simulink model "ExampleMotive"  (Simulink 8.5)
settings: Solver=ode1  StartTime=0.0  StopTime=inf  FixedStep=0.002  RelTol=1e-3
InitFcn:
  | fig_h = figure;
  | ax_h = axes;
  | set(ax_h,'Xlim',[-100 100],'YLim',[-100 100])
settings Model: Creator=adm-drone  LastModifiedBy=jitesh_esb201  ExtModeTrigDuration=5000
settings SolverCC: PositivePriorityOrder=on
settings DataIOCC: SignalLoggingSaveFormat=Dataset
settings OptimizationCC: ExpressionDepthLimit=128
settings DebuggingCC: SolverPrmCheckMsg=warning  FcnCallInpInsideContextMsg=EnableAllAsError
settings RTWCC: SystemTargetFile=quarc_win64.tlc  TemplateMakefile=quarc_default_tmf  Description=QUARC Win64 Target
settings STFCustomTargetCC: TargetPreCompLibLocation=C:\PROGRA~3\QUARC\lib\2013a\win64\release  GeneratePreprocessorConditionals=Disable all  CombineOutputUpdateFcns=on  CPPClassGenCompliant=on  GRTInterface=off  SystemTargetFile=quarc_win64.tlc
settings GRTTargetCC: TargetPreCompLibLocation=C:\PROGRA~3\QUARC\lib\2013a\win64\release  ParMdlRefBuildCompliant=off  CompOptLevelCompliant=off  ConcurrentExecutionCompliant=off  CombineOutputUpdateFcns=on  MatFileLogging=off  GRTInterface=off  ExtMode=on  ExtModeMexFile=quarc_comm

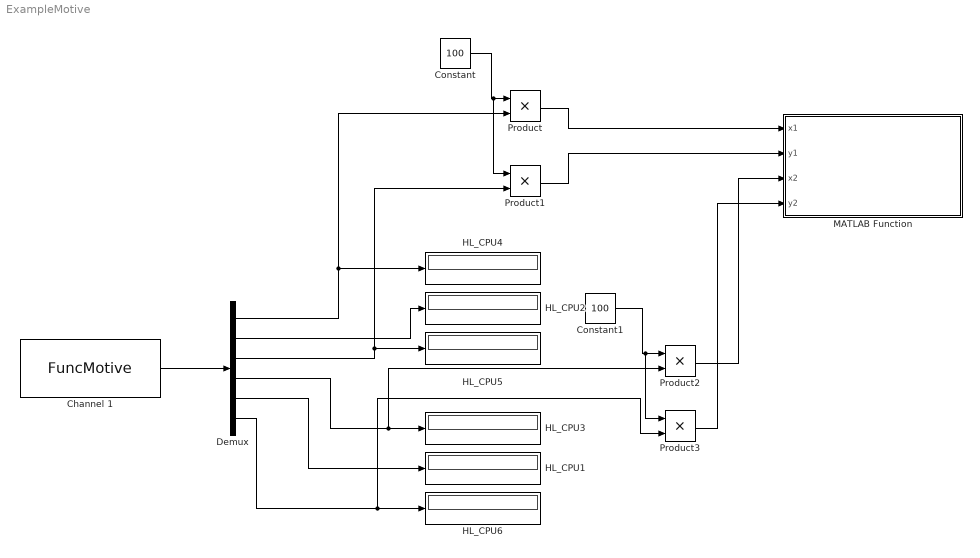
== system ExampleMotive ==
  Channel 1 : M-S-Function  FunctionName=FuncMotive  Parameters=1
  Constant : Constant  Value=100
  Constant1 : Constant  Value=100
  Demux : Demux  Outputs=6
  HL_CPU{1..6} (6 alike) : Display
  MATLAB Function : MATLAB Function  TreatAsAtomicUnit=on
  Product{,1..3} (4 alike) : Product
  wires:
  Channel 1/1 -> Demux/1
  Demux/1 -> Product/2, HL_CPU4/1
  Demux/2 -> HL_CPU2/1
  Demux/3 -> HL_CPU5/1, Product1/2
  Product/1 -> MATLAB Function/1(x1)
  Product1/1 -> MATLAB Function/2(y1)
  Constant/1 -> Product1/1, Product/1
  Demux/4 -> Product2/2, HL_CPU3/1
  Demux/5 -> HL_CPU1/1
  Demux/6 -> Product3/2, HL_CPU6/1
  Constant1/1 -> Product3/1, Product2/1
  Product2/1 -> MATLAB Function/3(x2)
  Product3/1 -> MATLAB Function/4(y2)

== matlab function MATLAB Function ==
  data: x1 input double; y1 input double; x2 input double; y2 input double
function plot_game(x1,y1,x2,y2)
%#codegen

coder.extrinsic('plot')
plot(x1,y1,'s','Markersize',8,'MarkerFaceColor','g','erasemode','xor');
hold
plot(x2,y2,'s','Markersize',8,'MarkerFaceColor','r','erasemode','xor');
set(gca,'XLim',[-100 100],'Ylim',[-100 100]) % or whatever axes limits you want
grid on;
xlabel(' x distance - cms');
ylabel(' y distance - cms');
